simulink model "admire_rtw"  (Simulink 3.00)
settings: Solver=ode3  SolverMode=SingleTasking  StartTime=0.0  StopTime=3000  FixedStep=0.01  RelTol=1e-3  AbsTol=1e-6
values from neighbouring files (symbols this model uses):
  x0 = [ max(eyp,zeros(n,1));max(-eyp,zeros(n,1));zeros(2*m,1)]    [LPwrap.m]
undefined symbols (not defined in the file or in its folder): dalpha_err, dalt_err, dbeta_err, dCl_beta, dCl_dai, dCl_day, dCl_dr, dCl_p, dCl_r, dCm_alpha, dCm_dei, dCm_dey, dCm_dne, dCm_q, dCn_beta, dCn_dna, dCn_dr, dCn_p, dCn_r, dCn_zero, ddc_bw, ddc_rate, ddei_bw, ddei_rate, ddey_bw, ddey_rate, ddle_bw, ddle_rate, ddr_bw, ddr_rate, dIxx, dIxz, dIyy, dIzz, dmass, dVt_err, dxcg, dycg, dzcg, rlimit_c, rlimit_ie, rlimit_le, rlimit_oe, rlimit_r, tasktype, tasktype_pitch, u0corr, u0fcs, u0new, x0diff, y0bare
libraries: simulink_extras x27, simulink3 x22
(part 2 of 2)

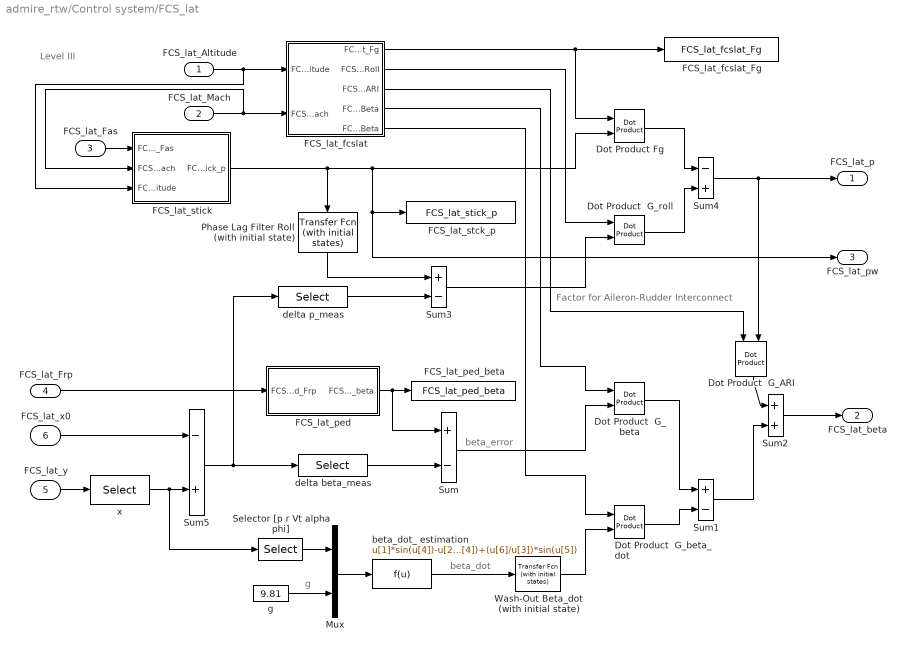
== system admire_rtw/Control system/FCS_lat ==
  note: g
  note: beta_dot
  note: beta_error
  note: Level III
  note: Factor for Aileron-Rudder
      | Interconnect
  "FCS_lat_Altitude " : Inport  Port=1  PortWidth=-1  SampleTime=-1  DataType=auto
      settings: SignalType=auto
  "FCS_lat_Mach " : Inport  Port=2  PortWidth=-1  SampleTime=-1  DataType=auto
      settings: SignalType=auto
  FCS_lat_Fas : Inport  Port=3  PortWidth=-1  SampleTime=-1  DataType=auto
      settings: SignalType=auto
  FCS_lat_Frp : Inport  Port=4  PortWidth=-1  SampleTime=-1  DataType=auto
      settings: SignalType=auto
  "FCS_lat_y " : Inport  Port=5  PortWidth=-1  SampleTime=-1  DataType=auto
      settings: SignalType=auto
  FCS_lat_x0 : Inport  Port=6  PortWidth=-1  SampleTime=-1  DataType=auto
      settings: SignalType=auto
  "  x" : Selector  Elements=[1:12]  InputPortWidth=28
  Dot Product Fg : simulink3/Math/Dot Product
  Dot Product  G_ARI : simulink3/Math/Dot Product  Orientation=down
  Dot Product  G_beta : simulink3/Math/Dot Product
  Dot Product  G_beta_dot : simulink3/Math/Dot Product
  Dot Product  G_roll : simulink3/Math/Dot Product
  FCS_lat_fcslat : Subsystem
      mask Display: disp('Calc of lateral\namplfication\n factors')
  FCS_lat_fcslat_Fg : ToWorkspace  VariableName=FCS_lat_fcslat_Fg  SampleTime=-1  SaveFormat=Matrix
  FCS_lat_ped : Subsystem
      mask Display: disp('FCS lateral pedal\nforce N to beta rad')
  FCS_lat_ped_beta : ToWorkspace  VariableName=FCS_lat_ped_beta  SampleTime=-1  SaveFormat=Matrix
  FCS_lat_stck_p : ToWorkspace  VariableName=FCS_lat_stick_p  SampleTime=-1  SaveFormat=Matrix
  FCS_lat_stick : Subsystem
      mask Display: disp('FCS lateral stick\ngradient\n N to rad/s')
  Mux : Mux  Inputs=2
      settings: DisplayOption=none
  Phase Lag Filter Roll (with initial state) : simulink_extras/Additional Linear/Transfer Fcn (with initial states)  Orientation=down  N=[0 1]  D="[0.25  1]"  X0=x0(39)
  Selector [p r Vt alpha phi] : Selector  Elements=[4 6 1 2 9]  InputPortWidth=12
  Sum : Sum  Inputs=+-  SaturateOnIntegerOverflow=on
  Sum1 : Sum  Inputs=+-  SaturateOnIntegerOverflow=on
  Sum2 : Sum  Inputs=++  SaturateOnIntegerOverflow=on
  Sum3 : Sum  Inputs=+-  SaturateOnIntegerOverflow=on
  Sum4 : Sum  Inputs=-+  SaturateOnIntegerOverflow=on
  Sum5 : Sum  Inputs=-+  SaturateOnIntegerOverflow=on
  Wash-Out Beta_dot (with initial state) : simulink_extras/Additional Linear/Transfer Fcn (with initial states)  N=[5 0]  D="[5  1]"  X0=x0(40)
  beta_dot_ estimation : Fcn  Expr=u[1]*sin(u[4])-u[2]*cos(u[4])+(u[6]/u[3])*sin(u[5])
  delta beta_meas : Selector  Elements=3  InputPortWidth=12
  delta p_meas : Selector  Elements=4  InputPortWidth=12
  g : Constant  Value=9.81
  "FCS_lat_p " : Outport  Port=1  InitialOutput=0
  "FCS_lat_beta " : Outport  Port=2  InitialOutput=0
  FCS_lat_pw : Outport  Port=3  InitialOutput=0
  wires:
  FCS_lat_Fas/1 -> FCS_lat_stick/1("FCS_lat_stick_Fas ")
  Phase Lag Filter Roll (with initial state)/1 -> Sum3/1
  delta p_meas/1 -> Sum3/2
  Mux/1 -> beta_dot_ estimation/1
  Selector [p r Vt alpha phi]/1 -> Mux/1
  g/1 -> Mux/2
  beta_dot_ estimation/1 -> Wash-Out Beta_dot (with initial state)/1
  Sum3/1 -> Dot Product  G_roll/2
  Dot Product  G_roll/1 -> Sum4/2
  Dot Product Fg/1 -> Sum4/1
  Wash-Out Beta_dot (with initial state)/1 -> Dot Product  G_beta_dot/2
  Dot Product  G_beta/1 -> Sum1/1
  Dot Product  G_beta_dot/1 -> Sum1/2
  Sum4/1 -> Dot Product  G_ARI/2, "FCS_lat_p "/1
  Dot Product  G_ARI/1 -> Sum2/1
  Sum2/1 -> "FCS_lat_beta "/1
  Sum1/1 -> Sum2/2
  FCS_lat_stick/1(FCS_lat_stick_p) -> Phase Lag Filter Roll (with initial state)/1, Dot Product Fg/2, FCS_lat_pw/1, FCS_lat_stck_p/1
  FCS_lat_fcslat/2(FCS_lat_fcslat_GRoll) -> Dot Product  G_roll/1
  FCS_lat_fcslat/3(FCS_lat_fcslat_GARI) -> Dot Product  G_ARI/1
  FCS_lat_fcslat/4(FCS_lat_fcslat_GBeta) -> Dot Product  G_beta/1
  FCS_lat_fcslat/5(FCS_lat_fcslat_dGBeta) -> Dot Product  G_beta_dot/1
  delta beta_meas/1 -> Sum/2
  Sum/1 -> Dot Product  G_beta/2
  FCS_lat_Frp/1 -> FCS_lat_ped/1(FCS_lat_ped_Frp)
  "FCS_lat_Altitude "/1 -> FCS_lat_fcslat/1(FCS_lat_fcslat_Altitude), FCS_lat_stick/3("FCS_lat_stick_Altitude ")
  "FCS_lat_Mach "/1 -> FCS_lat_stick/2("FCS_lat_stick_Mach "), FCS_lat_fcslat/2(FCS_lat_fcslat_Mach)
  "FCS_lat_y "/1 -> "  x"/1
  FCS_lat_x0/1 -> Sum5/1
  "  x"/1 -> Sum5/2, Selector [p r Vt alpha phi]/1
  Sum5/1 -> delta beta_meas/1, delta p_meas/1
  FCS_lat_fcslat/1(FCS_lat_fcslat_Fg) -> Dot Product Fg/1, FCS_lat_fcslat_Fg/1
  FCS_lat_ped/1(FCS_lat_ped_beta) -> FCS_lat_ped_beta/1, Sum/1

== system admire_rtw/Control system/FCS_long ==
  note: Level III
  note: q_feedback
      | to integrator
  note: Nz_feedback
      | to integrator
  note: [rad]
  "FCS_long_pw " : Inport  Port=1  PortWidth=-1  SampleTime=-1  DataType=auto
      settings: SignalType=auto
  "FCS_long_Altitude " : Inport  Port=2  PortWidth=-1  SampleTime=-1  DataType=auto
      settings: SignalType=auto
  FCS_long_Mach : Inport  Port=3  PortWidth=-1  SampleTime=-1  DataType=auto
      settings: SignalType=auto
  FCS_long_y : Inport  Port=4  PortWidth=-1  SampleTime=-1  DataType=auto
      settings: SignalType=auto
  FCS_long_Fes : Inport  Port=5  PortWidth=-1  SampleTime=-1  DataType=auto
      settings: SignalType=auto
  "FCS_long_Vt " : Inport  Port=6  PortWidth=-1  SampleTime=-1  DataType=auto
      settings: SignalType=auto
  FCS_long_Nz : Subsystem
      mask Display: disp('FCS_long_Nz')
  FCS_long_qVt : Subsystem
      mask Display: disp('FCS_long_qVt')
  Integrator : Integrator  ExternalReset=none  InitialConditionSource=internal  InitialCondition=x0(38)  LimitOutput=off  UpperSaturationLimit=inf  LowerSaturationLimit=-inf  ShowSaturationPort=off  ShowStatePort=off  AbsoluteTolerance=auto
  Sum : Sum  Inputs=+++  SaturateOnIntegerOverflow=on
  Sum1 : Sum  Inputs=++  SaturateOnIntegerOverflow=on
  FCS_long_x0 : Outport  Port=1  InitialOutput=0
  FCS_long_q : Outport  Port=2  InitialOutput=0
  FCS_long_tss : Outport  Port=3  InitialOutput=0
  wires:
  "FCS_long_Vt "/1 -> FCS_long_qVt/3(FCS_long_qVt_Vt)
  FCS_long_Mach/1 -> FCS_long_qVt/2(FCS_long_qVt_Mach), FCS_long_Nz/2("FCS_long_Nz_Mach ")
  FCS_long_y/1 -> FCS_long_qVt/4(FCS_long_qVt_y), FCS_long_Nz/3(FCS_long_Nz_y)
  FCS_long_qVt/1(FCS_long_qVt_x0) -> FCS_long_x0/1, FCS_long_Nz/5(FCS_long_Nz_x0)
  FCS_long_Fes/1 -> FCS_long_qVt/5(FCS_long_qVt_Fes), FCS_long_Nz/4(FCS_long_Nz_Fes)
  "FCS_long_pw "/1 -> FCS_long_qVt/6("FCS_long_qVt_pw ")
  FCS_long_qVt/2(FCS_long_qVt_tss) -> FCS_long_tss/1
  FCS_long_qVt/3(FCS_long_qVt_q) -> Sum/1
  FCS_long_Nz/1(FCS_long_Nz_control) -> Sum/2
  "FCS_long_Altitude "/1 -> FCS_long_qVt/1(FCS_long_qVt_Altitude), FCS_long_Nz/1("FCS_long_Nz_Altitude ")
  Sum/1 -> FCS_long_q/1
  FCS_long_qVt/4(FCS_long_qVt_fbi) -> Sum1/1
  FCS_long_Nz/2(FCS_long_Nz_fbi) -> Sum1/2
  Integrator/1 -> Sum/3
  Sum1/1 -> Integrator/1

== system admire_rtw/FCS_ae_rl/FCS_ae_rl_lc ==
  note: Level V
  FCS_ae_rl_lc_dlc : Inport  Port=1  PortWidth=-1  SampleTime=-1  DataType=auto
      settings: SignalType=auto
  RL2 : RateLimiter  RisingSlewLimit=rlimit_c+ddc_rate  FallingSlewLimit=-rlimit_c-ddc_rate
  dlc_actuator (with initial state) : simulink_extras/Additional Linear/Transfer Fcn (with initial states)  N=[1]  D="[0.05+ddc_bw  1]"  X0=x0(2)
  dlc_l : ToWorkspace  VariableName=dlc_l  SampleTime=0  SaveFormat=Matrix
  dlc_r : ToWorkspace  VariableName=dlc_r  SampleTime=0  SaveFormat=Matrix
  FCS_ae_rl_lc_dlc_out : Outport  Port=1  InitialOutput=0
  wires:
  FCS_ae_rl_lc_dlc/1 -> dlc_l/1, RL2/1
  dlc_actuator (with initial state)/1 -> FCS_ae_rl_lc_dlc_out/1
  RL2/1 -> dlc_r/1, dlc_actuator (with initial state)/1

== system admire_rtw/FCS_ae_rl/FCS_ae_rl_le ==
  note: Level V
  FCS_ae_rl_le_dle : Inport  Port=1  PortWidth=-1  SampleTime=-1  DataType=auto
      settings: SignalType=auto
  RL2 : RateLimiter  RisingSlewLimit=rlimit_le+ddle_rate  FallingSlewLimit=-rlimit_le-ddle_rate
  dle_actuator (with initial state) : simulink_extras/Additional Linear/Transfer Fcn (with initial states)  N=[1]  D="[0.05+ddle_bw  1]"  X0=x0(8)
  dle_l : ToWorkspace  VariableName=dle_l  SampleTime=0  SaveFormat=Matrix
  dle_r : ToWorkspace  VariableName=dle_r  SampleTime=0  SaveFormat=Matrix
  FCS_ae_rl_le_dle_out : Outport  Port=1  InitialOutput=0
  wires:
  FCS_ae_rl_le_dle/1 -> dle_l/1, RL2/1
  dle_actuator (with initial state)/1 -> FCS_ae_rl_le_dle_out/1
  RL2/1 -> dle_r/1, dle_actuator (with initial state)/1

== system admire_rtw/FCS_ae_rl/FCS_ae_rl_lie ==
  note: Level V
  FCS_ae_rl_lie_dlie : Inport  Port=1  PortWidth=-1  SampleTime=-1  DataType=auto
      settings: SignalType=auto
  RL2 : RateLimiter  RisingSlewLimit=rlimit_ie+ddei_rate  FallingSlewLimit=-rlimit_ie-ddei_rate
  dlie_actuator (with initial state) : simulink_extras/Additional Linear/Transfer Fcn (with initial states)  N=[1]  D="[0.05+ddei_bw  1]"  X0=x0(5)
  dlie_l : ToWorkspace  VariableName=dlie_l  SampleTime=0  SaveFormat=Matrix
  dlie_r : ToWorkspace  VariableName=dlie_r  SampleTime=0  SaveFormat=Matrix
  FCS_ae_rl_lie_dlie_out : Outport  Port=1  InitialOutput=0
  wires:
  dlie_actuator (with initial state)/1 -> FCS_ae_rl_lie_dlie_out/1
  FCS_ae_rl_lie_dlie/1 -> dlie_l/1, RL2/1
  RL2/1 -> dlie_actuator (with initial state)/1, dlie_r/1

== system admire_rtw/FCS_ae_rl/FCS_ae_rl_loe ==
  note: Level V
  FCS_ae_rl_loe_dloe : Inport  Port=1  PortWidth=-1  SampleTime=-1  DataType=auto
      settings: SignalType=auto
  RL2 : RateLimiter  RisingSlewLimit=rlimit_oe+ddey_rate  FallingSlewLimit=-rlimit_oe-ddey_rate
  dloe_actuator (with initial state) : simulink_extras/Additional Linear/Transfer Fcn (with initial states)  N=[1]  D="[0.05+ddey_bw  1]"  X0=x0(6)
  dloe_l : ToWorkspace  VariableName=dloe_l  SampleTime=0  SaveFormat=Matrix
  dloe_r : ToWorkspace  VariableName=dloe_r  SampleTime=0  SaveFormat=Matrix
  FCS_ae_rl_loe_dloe_out : Outport  Port=1  InitialOutput=0
  wires:
  FCS_ae_rl_loe_dloe/1 -> dloe_l/1, RL2/1
  dloe_actuator (with initial state)/1 -> FCS_ae_rl_loe_dloe_out/1
  RL2/1 -> dloe_r/1, dloe_actuator (with initial state)/1

== system admire_rtw/FCS_ae_rl/FCS_ae_rl_r ==
  note: Level V
  FCS_ae_rl_r_dr : Inport  Port=1  PortWidth=-1  SampleTime=-1  DataType=auto
      settings: SignalType=auto
  RL2 : RateLimiter  RisingSlewLimit=rlimit_r+ddr_rate  FallingSlewLimit=-rlimit_r-ddr_rate
  dr_actuator (with initial state) : simulink_extras/Additional Linear/Transfer Fcn (with initial states)  N=[1]  D="[0.05+ddr_bw  1]"  X0=x0(7)
  dr_l : ToWorkspace  VariableName=dr_l  SampleTime=0  SaveFormat=Matrix
  dr_r : ToWorkspace  VariableName=dr_r  SampleTime=0  SaveFormat=Matrix
  FCS_ae_rl_r_dr_out : Outport  Port=1  InitialOutput=0
  wires:
  dr_actuator (with initial state)/1 -> FCS_ae_rl_r_dr_out/1
  FCS_ae_rl_r_dr/1 -> dr_l/1, RL2/1
  RL2/1 -> dr_actuator (with initial state)/1, dr_r/1

== system admire_rtw/FCS_ae_rl/FCS_ae_rl_rc ==
  note: Level V
  FCS_ae_rl_rc_drc : Inport  Port=1  PortWidth=-1  SampleTime=-1  DataType=auto
      settings: SignalType=auto
  RL2 : RateLimiter  RisingSlewLimit=rlimit_c+ddc_rate  FallingSlewLimit=-rlimit_c-ddc_rate
  drc_actuator (with initial state) : simulink_extras/Additional Linear/Transfer Fcn (with initial states)  N=[1]  D="[0.05+ddc_bw  1]"  X0=x0(1)
  drc_l : ToWorkspace  VariableName=drc_l  SampleTime=0  SaveFormat=Matrix
  drc_r : ToWorkspace  VariableName=drc_r  SampleTime=0  SaveFormat=Matrix
  FCS_ae_rl_rc_drc_out : Outport  Port=1  InitialOutput=0
  wires:
  drc_actuator (with initial state)/1 -> FCS_ae_rl_rc_drc_out/1
  FCS_ae_rl_rc_drc/1 -> drc_l/1, RL2/1
  RL2/1 -> drc_actuator (with initial state)/1, drc_r/1

== system admire_rtw/FCS_ae_rl/FCS_ae_rl_rie ==
  note: Level V
  FCS_ae_rl_rie_drie : Inport  Port=1  PortWidth=-1  SampleTime=-1  DataType=auto
      settings: SignalType=auto
  RL2 : RateLimiter  RisingSlewLimit=rlimit_ie+ddei_rate  FallingSlewLimit=-rlimit_ie-ddei_rate
  drie_actuator (with initial state) : simulink_extras/Additional Linear/Transfer Fcn (with initial states)  N=[1]  D="[0.05+ddei_bw  1]"  X0=x0(4)
  drie_l : ToWorkspace  VariableName=drie_l  SampleTime=0  SaveFormat=Matrix
  drie_r : ToWorkspace  VariableName=drie_r  SampleTime=0  SaveFormat=Matrix
  FCS_ae_rl_rie_drie_out : Outport  Port=1  InitialOutput=0
  wires:
  FCS_ae_rl_rie_drie/1 -> drie_l/1, RL2/1
  drie_actuator (with initial state)/1 -> FCS_ae_rl_rie_drie_out/1
  RL2/1 -> drie_r/1, drie_actuator (with initial state)/1

== system admire_rtw/FCS_ae_rl/FCS_ae_rl_roe ==
  note: Level V
  FCS_ae_rl_roe_droe : Inport  Port=1  PortWidth=-1  SampleTime=-1  DataType=auto
      settings: SignalType=auto
  RL2 : RateLimiter  RisingSlewLimit=rlimit_oe+ddey_rate  FallingSlewLimit=-rlimit_oe-ddey_rate
  droe_actuator (with initial state) : simulink_extras/Additional Linear/Transfer Fcn (with initial states)  N=[1]  D="[0.05+ddey_bw  1]"  X0=x0(3)
  droe_l : ToWorkspace  VariableName=droe_l  SampleTime=0  SaveFormat=Matrix
  droe_r : ToWorkspace  VariableName=droe_r  SampleTime=0  SaveFormat=Matrix
  FCS_ae_rl_roe_droe_out : Outport  Port=1  InitialOutput=0
  wires:
  droe_actuator (with initial state)/1 -> FCS_ae_rl_roe_droe_out/1
  FCS_ae_rl_roe_droe/1 -> droe_l/1, RL2/1
  RL2/1 -> droe_actuator (with initial state)/1, droe_r/1

== system admire_rtw/Aircraft response/Sensor models/Subsystem To Gain-Scheduling ==
  note: Level III
  Vt [m/s] : Inport  Port=1  PortWidth=-1  SampleTime=-1  DataType=auto
      settings: SignalType=auto
  alt [m] : Inport  Port=2  PortWidth=-1  SampleTime=-1  DataType=auto
      settings: SignalType=auto
  S-Function : S-Function  FunctionName=machno  PortCounts=[]  SFunctionModules=''
  Mach : Outport  Port=1
  tag scope: Altitude=global, Mach=global
  wires:
  alt [m]/1 -> [Altitude], S-Function/2
  Vt [m/s]/1 -> S-Function/1
  S-Function/1 -> [Mach], Mach/1

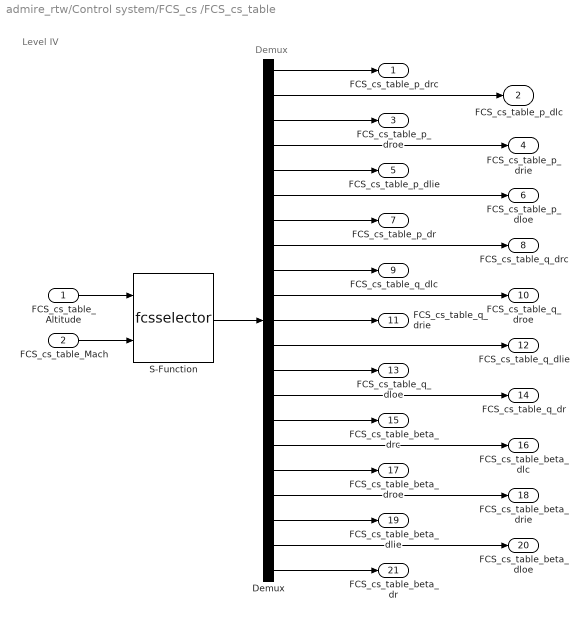
== system admire_rtw/Control system/FCS_cs /FCS_cs_table ==
  note: Level IV
  note: Demux
  FCS_cs_table_Altitude : Inport  Port=1  PortWidth=-1  SampleTime=-1  DataType=auto
      settings: SignalType=auto
  FCS_cs_table_Mach : Inport  Port=2  PortWidth=-1  SampleTime=-1  DataType=auto
      settings: SignalType=auto
  Demux : Demux  Outputs=21
  S-Function : S-Function  FunctionName=fcsselector  PortCounts=[]  SFunctionModules=''
  FCS_cs_table_p_drc : Outport  Port=1
  FCS_cs_table_p_dlc : Outport  Port=2
  FCS_cs_table_p_droe : Outport  Port=3
  FCS_cs_table_p_drie : Outport  Port=4
  FCS_cs_table_p_dlie : Outport  Port=5
  FCS_cs_table_p_dloe : Outport  Port=6
  FCS_cs_table_p_dr : Outport  Port=7
  FCS_cs_table_q_drc : Outport  Port=8
  FCS_cs_table_q_dlc : Outport  Port=9
  FCS_cs_table_q_droe : Outport  Port=10
  FCS_cs_table_q_drie : Outport  Port=11
  FCS_cs_table_q_dlie : Outport  Port=12
  FCS_cs_table_q_dloe : Outport  Port=13
  FCS_cs_table_q_dr : Outport  Port=14
  FCS_cs_table_beta_drc : Outport  Port=15
  FCS_cs_table_beta_dlc : Outport  Port=16
  FCS_cs_table_beta_droe : Outport  Port=17
  FCS_cs_table_beta_drie : Outport  Port=18
  FCS_cs_table_beta_dlie : Outport  Port=19
  FCS_cs_table_beta_dloe : Outport  Port=20
  FCS_cs_table_beta_dr : Outport  Port=21
  wires:
  FCS_cs_table_Altitude/1 -> S-Function/1
  FCS_cs_table_Mach/1 -> S-Function/2
  S-Function/1 -> Demux/1
  Demux/3 -> FCS_cs_table_p_droe/1
  Demux/5 -> FCS_cs_table_p_dlie/1
  Demux/7 -> FCS_cs_table_p_dr/1
  Demux/9 -> FCS_cs_table_q_dlc/1
  Demux/11 -> FCS_cs_table_q_drie/1
  Demux/13 -> FCS_cs_table_q_dloe/1
  Demux/15 -> FCS_cs_table_beta_drc/1
  Demux/17 -> FCS_cs_table_beta_droe/1
  Demux/19 -> FCS_cs_table_beta_dlie/1
  Demux/21 -> FCS_cs_table_beta_dr/1
  Demux/2 -> FCS_cs_table_p_dlc/1
  Demux/4 -> FCS_cs_table_p_drie/1
  Demux/6 -> FCS_cs_table_p_dloe/1
  Demux/8 -> FCS_cs_table_q_drc/1
  Demux/10 -> FCS_cs_table_q_droe/1
  Demux/12 -> FCS_cs_table_q_dlie/1
  Demux/16 -> FCS_cs_table_beta_dlc/1
  Demux/18 -> FCS_cs_table_beta_drie/1
  Demux/20 -> FCS_cs_table_beta_dloe/1
  Demux/14 -> FCS_cs_table_q_dr/1
  Demux/1 -> FCS_cs_table_p_drc/1

== system admire_rtw/Control system/FCS_lat/FCS_lat_fcslat ==
  note: Level IV
  note: S-function
  FCS_lat_fcslat_Altitude : Inport  Port=1  PortWidth=-1  SampleTime=-1  DataType=auto
      settings: SignalType=auto
  FCS_lat_fcslat_Mach : Inport  Port=2  PortWidth=-1  SampleTime=-1  DataType=auto
      settings: SignalType=auto
  S-Function : S-Function  FunctionName=fcslateral  PortCounts=[]  SFunctionModules=''
  FCS_lat_fcslat_Fg : Outport  Port=1
  FCS_lat_fcslat_GRoll : Outport  Port=2
  FCS_lat_fcslat_GARI : Outport  Port=3
  FCS_lat_fcslat_GBeta : Outport  Port=4
  FCS_lat_fcslat_dGBeta : Outport  Port=5
  wires:
  FCS_lat_fcslat_Altitude/1 -> S-Function/1
  FCS_lat_fcslat_Mach/1 -> S-Function/2
  S-Function/1 -> FCS_lat_fcslat_Fg/1
  S-Function/2 -> FCS_lat_fcslat_GBeta/1
  S-Function/3 -> FCS_lat_fcslat_dGBeta/1
  S-Function/4 -> FCS_lat_fcslat_GARI/1
  S-Function/5 -> FCS_lat_fcslat_GRoll/1

== system admire_rtw/Control system/FCS_lat/FCS_lat_ped ==
  note: Level IV
  FCS_lat_ped_Frp : Inport  Port=1  PortWidth=-1  SampleTime=-1  DataType=auto
      settings: SignalType=auto
  Degrees to Radians : simulink_extras/Transformations/Degrees to Radians
  Look-Up Table Frp gradient : Lookup  InputValues=[-200 0 200]  OutputValues=[5 0 -5]
  Saturation : Saturate  UpperLimit=200  LowerLimit=-200
  FCS_lat_ped_beta : Outport  Port=1
  wires:
  Saturation/1 -> Look-Up Table Frp gradient/1
  FCS_lat_ped_Frp/1 -> Saturation/1
  Degrees to Radians/1 -> FCS_lat_ped_beta/1
  Look-Up Table Frp gradient/1 -> Degrees to Radians/1

== system admire_rtw/Control system/FCS_lat/FCS_lat_stick ==
  note: Level IV
  "FCS_lat_stick_Fas " : Inport  Port=1  PortWidth=-1  SampleTime=-1  DataType=auto
      settings: SignalType=auto
  "FCS_lat_stick_Mach " : Inport  Port=2  PortWidth=-1  SampleTime=-1  DataType=auto
      settings: SignalType=auto
  "FCS_lat_stick_Altitude " : Inport  Port=3  PortWidth=-1  SampleTime=-1  DataType=auto
      settings: SignalType=auto
  Dead Zone  +- 3N : DeadZone  LowerValue=-3  UpperValue=3
  Degrees to Radians : simulink_extras/Transformations/Degrees to Radians
  Gain : Gain  Gain=180/80  SaturateOnIntegerOverflow=on
  Saturation : Saturate  UpperLimit=80  LowerLimit=-80
  Terminator : Terminator
  Terminator 2 : Terminator
  FCS_lat_stick_p : Outport  Port=1
  wires:
  Degrees to Radians/1 -> FCS_lat_stick_p/1
  Saturation/1 -> Gain/1
  Gain/1 -> Degrees to Radians/1
  "FCS_lat_stick_Mach "/1 -> Terminator/1
  "FCS_lat_stick_Altitude "/1 -> Terminator 2/1
  Dead Zone  +- 3N/1 -> Saturation/1
  "FCS_lat_stick_Fas "/1 -> Dead Zone  +- 3N/1

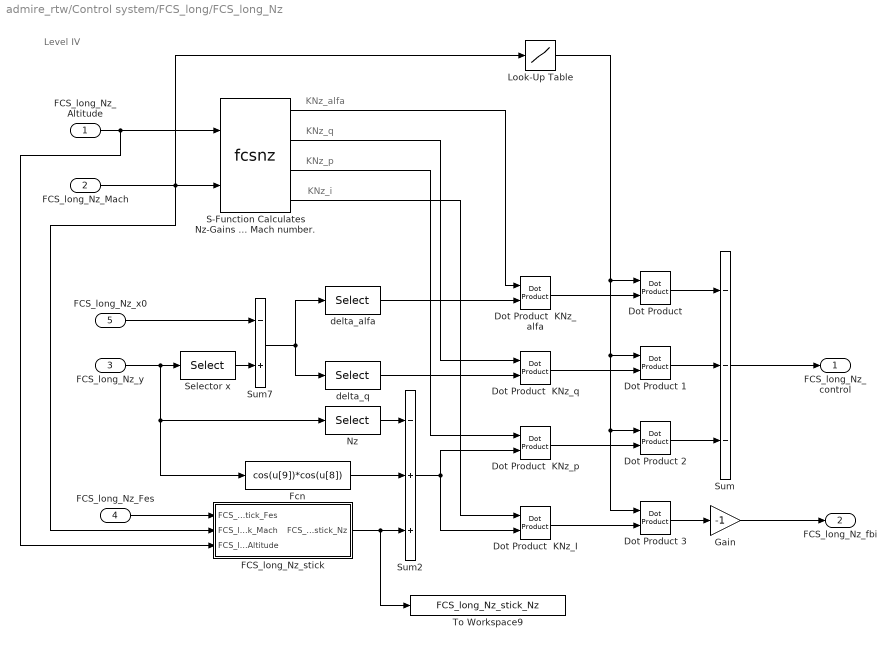
== system admire_rtw/Control system/FCS_long/FCS_long_Nz ==
  note: KNz_alfa
  note: KNz_q
  note: KNz_p
  note: KNz_i
  note: Level IV
  "FCS_long_Nz_Altitude " : Inport  Port=1  PortWidth=-1  SampleTime=-1  DataType=auto
      settings: SignalType=auto
  "FCS_long_Nz_Mach " : Inport  Port=2  PortWidth=-1  SampleTime=-1  DataType=auto
      settings: SignalType=auto
  FCS_long_Nz_y : Inport  Port=3  PortWidth=-1  SampleTime=-1  DataType=auto
      settings: SignalType=auto
  FCS_long_Nz_Fes : Inport  Port=4  PortWidth=-1  SampleTime=-1  DataType=auto
      settings: SignalType=auto
  FCS_long_Nz_x0 : Inport  Port=5  PortWidth=-1  SampleTime=-1  DataType=auto
      settings: SignalType=auto
  Dot Product {,1..3} (4 alike) : simulink3/Math/Dot Product
  Dot Product  KNz_I : simulink3/Math/Dot Product
  Dot Product  KNz_alfa : simulink3/Math/Dot Product
  Dot Product  KNz_p : simulink3/Math/Dot Product
  Dot Product  KNz_q : simulink3/Math/Dot Product
  FCS_long_Nz_stick : Subsystem
      mask Display: disp('FCS_long_Nz_stick')
  Fcn : Fcn  Expr=cos(u[9])*cos(u[8])
  Gain : Gain  Gain=-1  SaturateOnIntegerOverflow=on
  Look-Up Table : Lookup  InputValues=[0 0.58 0.62 2.5]  OutputValues=[0 0 1 1]
  Nz : Selector  Elements=19  InputPortWidth=28
  S-Function Calculates Nz-Gains as a function of altitude and Mach number. : S-Function  FunctionName=fcsnz  PortCounts=[]  SFunctionModules=''
  Selector x : Selector  Elements=[1:12]  InputPortWidth=28
  Sum : Sum  Inputs=---  SaturateOnIntegerOverflow=on
  Sum2 : Sum  Inputs=-++  SaturateOnIntegerOverflow=on
  Sum7 : Sum  Inputs=-+  SaturateOnIntegerOverflow=on
  To Workspace9 : ToWorkspace  VariableName=FCS_long_Nz_stick_Nz  SampleTime=-1  SaveFormat=Matrix
  delta_alfa : Selector  Elements=2  InputPortWidth=12
  delta_q : Selector  Elements=5  InputPortWidth=12
  FCS_long_Nz_control : Outport  Port=1
  FCS_long_Nz_fbi : Outport  Port=2
  wires:
  Nz/1 -> Sum2/1
  FCS_long_Nz_Fes/1 -> FCS_long_Nz_stick/1("FCS_long_Nz_stick_Fes ")
  Selector x/1 -> Sum7/2
  FCS_long_Nz_x0/1 -> Sum7/1
  Sum7/1 -> delta_alfa/1, delta_q/1
  FCS_long_Nz_y/1 -> Selector x/1, Nz/1, Fcn/1
  "FCS_long_Nz_Mach "/1 -> S-Function Calculates Nz-Gains as a function of altitude and Mach number./2, Look-Up Table/1, FCS_long_Nz_stick/2(FCS_long_Nz_stick_Mach)
  Sum2/1 -> Dot Product  KNz_p/2, Dot Product  KNz_I/2
  S-Function Calculates Nz-Gains as a function of altitude and Mach number./4 -> Dot Product  KNz_I/1
  delta_alfa/1 -> Dot Product  KNz_alfa/2
  delta_q/1 -> Dot Product  KNz_q/2
  S-Function Calculates Nz-Gains as a function of altitude and Mach number./3 -> Dot Product  KNz_p/1
  S-Function Calculates Nz-Gains as a function of altitude and Mach number./2 -> Dot Product  KNz_q/1
  S-Function Calculates Nz-Gains as a function of altitude and Mach number./1 -> Dot Product  KNz_alfa/1
  "Dot Product "/1 -> Sum/1
  Dot Product  KNz_alfa/1 -> "Dot Product "/2
  Dot Product 1/1 -> Sum/2
  Dot Product  KNz_q/1 -> Dot Product 1/2
  Look-Up Table/1 -> "Dot Product "/1, Dot Product 1/1, Dot Product 2/1, Dot Product 3/1
  Dot Product 2/1 -> Sum/3
  Dot Product  KNz_p/1 -> Dot Product 2/2
  Dot Product  KNz_I/1 -> Dot Product 3/2
  Sum/1 -> FCS_long_Nz_control/1
  Gain/1 -> FCS_long_Nz_fbi/1
  Dot Product 3/1 -> Gain/1
  "FCS_long_Nz_Altitude "/1 -> S-Function Calculates Nz-Gains as a function of altitude and Mach number./1, FCS_long_Nz_stick/3("FCS_long_Nz_stick_Altitude ")
  FCS_long_Nz_stick/1(FCS_long_Nz_stick_Nz) -> To Workspace9/1, Sum2/3
  Fcn/1 -> Sum2/2

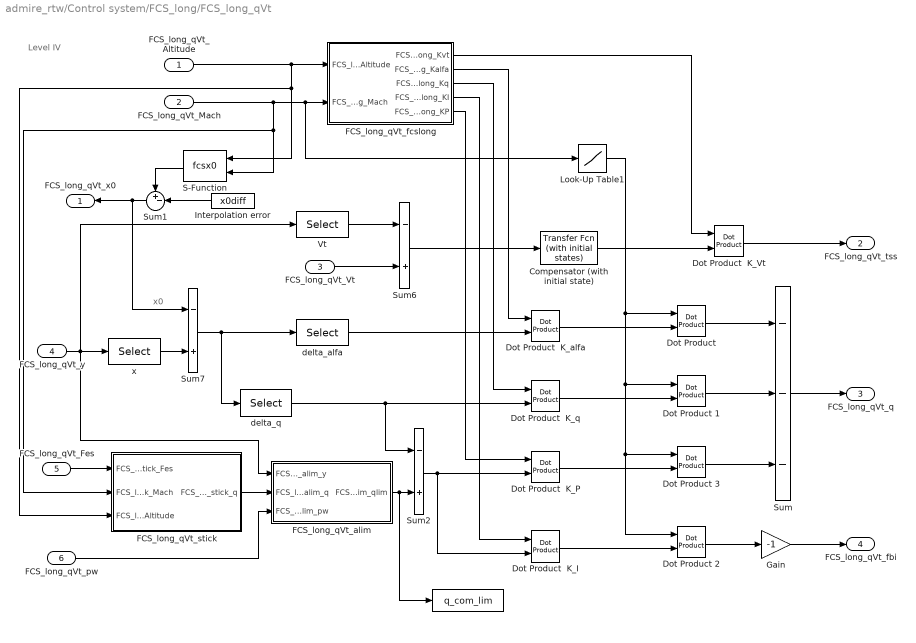
== system admire_rtw/Control system/FCS_long/FCS_long_qVt ==
  note: x0
  note: Level IV
  FCS_long_qVt_Altitude : Inport  Port=1  PortWidth=-1  SampleTime=-1  DataType=auto
      settings: SignalType=auto
  FCS_long_qVt_Mach : Inport  Port=2  PortWidth=-1  SampleTime=-1  DataType=auto
      settings: SignalType=auto
  FCS_long_qVt_Vt : Inport  Port=3  PortWidth=-1  SampleTime=-1  DataType=auto
      settings: SignalType=auto
  FCS_long_qVt_y : Inport  Port=4  PortWidth=-1  SampleTime=-1  DataType=auto
      settings: SignalType=auto
  FCS_long_qVt_Fes : Inport  Port=5  PortWidth=-1  SampleTime=-1  DataType=auto
      settings: SignalType=auto
  "FCS_long_qVt_pw " : Inport  Port=6  PortWidth=-1  SampleTime=-1  DataType=auto
      settings: SignalType=auto
  " " : ToWorkspace  VariableName=q_com_lim  SampleTime=-1  SaveFormat=Matrix
  Compensator (with initial state) : simulink_extras/Additional Linear/Transfer Fcn (with initial states)  N=[15 10]  D="[1  10]"  X0=x0(41)
  Dot Product {,1..3} (4 alike) : simulink3/Math/Dot Product
  Dot Product  K_I : simulink3/Math/Dot Product
  Dot Product  K_P : simulink3/Math/Dot Product
  Dot Product  K_Vt : simulink3/Math/Dot Product
  Dot Product  K_alfa : simulink3/Math/Dot Product
  Dot Product  K_q : simulink3/Math/Dot Product
  FCS_long_qVt_alim : Subsystem
      mask Display: disp('FCS_long_qVt_alim')
  FCS_long_qVt_fcslong : Subsystem
      mask Display: disp('FCS_long_qVt_fcslong')
  FCS_long_qVt_stick : Subsystem
      mask Display: disp('FCS_long_qVt_stick')
  Gain : Gain  Gain=-1  SaturateOnIntegerOverflow=on
  Interpolation error : Constant  Orientation=left  Value=x0diff
  Look-Up Table1 : Lookup  InputValues=[0 0.58 0.62 2.5]  OutputValues=[1 1 0 0]
  S-Function : S-Function  Orientation=left  FunctionName=fcsx0  PortCounts=[]  SFunctionModules=''
  Sum : Sum  Inputs=---  SaturateOnIntegerOverflow=on
  Sum1 : Sum  Orientation=left  Inputs=+-|  SaturateOnIntegerOverflow=on
  Sum2 : Sum  Inputs=-+  SaturateOnIntegerOverflow=on
  Sum6 : Sum  Inputs=-+  SaturateOnIntegerOverflow=on
  Sum7 : Sum  Inputs=-+  SaturateOnIntegerOverflow=on
  Vt : Selector  Elements=1  InputPortWidth=28
  delta_alfa : Selector  Elements=2  InputPortWidth=12
  delta_q : Selector  Elements=5  InputPortWidth=12
  x : Selector  Elements=[1:12]  InputPortWidth=28
  FCS_long_qVt_x0 : Outport  Orientation=left  Port=1
  FCS_long_qVt_tss : Outport  Port=2
  FCS_long_qVt_q : Outport  Port=3
  FCS_long_qVt_fbi : Outport  Port=4
  wires:
  FCS_long_qVt_fcslong/5(FCS_long_qVt_fcslong_KP) -> Dot Product  K_P/1
  FCS_long_qVt_Altitude/1 -> FCS_long_qVt_fcslong/1(FCS_long_qVt_fcslong_Altitude), FCS_long_qVt_stick/3("FCS_long_qVt_stick_Altitude "), S-Function/1
  FCS_long_qVt_Mach/1 -> FCS_long_qVt_stick/2("FCS_long_qVt_stick_Mach "), S-Function/2, FCS_long_qVt_fcslong/2(FCS_long_qVt_fcslong_Mach), Look-Up Table1/1
  delta_alfa/1 -> Dot Product  K_alfa/2
  x/1 -> Sum7/2
  Sum7/1 -> delta_alfa/1, delta_q/1
  delta_q/1 -> Dot Product  K_q/2, Sum2/1
  FCS_long_qVt_y/1 -> x/1, Vt/1, FCS_long_qVt_alim/1(FCS_long_qVt_alim_y)
  FCS_long_qVt_Fes/1 -> FCS_long_qVt_stick/1("FCS_long_qVt_stick_Fes ")
  FCS_long_qVt_alim/1(FCS_long_qVt_alim_qlim) -> Sum2/2, " "/1
  FCS_long_qVt_stick/1("FCS_long_qVt_stick_q ") -> FCS_long_qVt_alim/2("FCS_long_qVt_alim_q ")
  "FCS_long_qVt_pw "/1 -> FCS_long_qVt_alim/3(FCS_long_qVt_alim_pw)
  Compensator (with initial state)/1 -> Dot Product  K_Vt/2
  Dot Product  K_Vt/1 -> FCS_long_qVt_tss/1
  FCS_long_qVt_fcslong/1(FCS_long_qVt_fcslong_Kvt) -> Dot Product  K_Vt/1
  Sum2/1 -> Dot Product  K_P/2, Dot Product  K_I/2
  Dot Product  K_P/1 -> Dot Product 3/2
  Sum/1 -> FCS_long_qVt_q/1
  Dot Product  K_q/1 -> Dot Product 1/2
  Dot Product 1/1 -> Sum/2
  "Dot Product "/1 -> Sum/1
  Dot Product  K_alfa/1 -> "Dot Product "/2
  Look-Up Table1/1 -> "Dot Product "/1, Dot Product 1/1, Dot Product 3/1, Dot Product 2/1
  Sum6/1 -> Compensator (with initial state)/1
  Dot Product 3/1 -> Sum/3
  Gain/1 -> FCS_long_qVt_fbi/1
  Dot Product 2/1 -> Gain/1
  FCS_long_qVt_fcslong/3(FCS_long_qVt_fcslong_Kq) -> Dot Product  K_q/1
  FCS_long_qVt_fcslong/2(FCS_long_qVt_fcslong_Kalfa) -> Dot Product  K_alfa/1
  FCS_long_qVt_Vt/1 -> Sum6/2
  Vt/1 -> Sum6/1
  Dot Product  K_I/1 -> Dot Product 2/2
  FCS_long_qVt_fcslong/4(FCS_long_qVt_fcslong_KI) -> Dot Product  K_I/1
  Interpolation error/1 -> Sum1/2
  S-Function/1 -> Sum1/1
  Sum1/1 -> Sum7/1, FCS_long_qVt_x0/1

== system admire_rtw/Control system/FCS_long/FCS_long_Nz/FCS_long_Nz_stick ==
  note: Level V
  "FCS_long_Nz_stick_Fes " : Inport  Port=1  PortWidth=-1  SampleTime=-1  DataType=auto
      settings: SignalType=auto
  FCS_long_Nz_stick_Mach : Inport  Port=2  PortWidth=-1  SampleTime=-1  DataType=auto
      settings: SignalType=auto
  "FCS_long_Nz_stick_Altitude " : Inport  Port=3  PortWidth=-1  SampleTime=-1  DataType=auto
      settings: SignalType=auto
  Dead Zone  +- 1N : DeadZone  LowerValue=-1  UpperValue=1
  Gain : Gain  Gain=8/80  SaturateOnIntegerOverflow=on
  Saturation [-40,+80]   [Newton] : Saturate  UpperLimit=80  LowerLimit=-40
  Terminator : Terminator
  Terminator 2 : Terminator
  FCS_long_Nz_stick_Nz : Outport  Port=1
  wires:
  Saturation [-40,+80]   [Newton]/1 -> Gain/1
  Gain/1 -> FCS_long_Nz_stick_Nz/1
  "FCS_long_Nz_stick_Altitude "/1 -> Terminator 2/1
  FCS_long_Nz_stick_Mach/1 -> Terminator/1
  Dead Zone  +- 1N/1 -> Saturation [-40,+80]   [Newton]/1
  "FCS_long_Nz_stick_Fes "/1 -> Dead Zone  +- 1N/1

== system admire_rtw/Control system/FCS_long/FCS_long_qVt/FCS_long_qVt_alim ==
  note: Level V
  FCS_long_qVt_alim_y : Inport  Port=1  PortWidth=-1  SampleTime=-1  DataType=auto
      settings: SignalType=auto
  "FCS_long_qVt_alim_q " : Inport  Port=2  PortWidth=-1  SampleTime=-1  DataType=auto
      settings: SignalType=auto
  FCS_long_qVt_alim_pw : Inport  Port=3  PortWidth=-1  SampleTime=-1  DataType=auto
      settings: SignalType=auto
  FCS_long_qVt_alim_nega : Subsystem
      mask Display: disp('FCS_long_qVt_alim\nnegative alpha')
  FCS_long_qVt_alim_posa : Subsystem
      mask Display: disp('FCS_long_qVt_alim\npositive alpha')
  Logical Operator3 : Logic  Operator=OR  Inputs=3
  Logical Operator4 : Logic  Operator=NOT  Inputs=1
  Logical Operator5 : Logic  Orientation=up  Operator=NOT  Inputs=1
  Mach : Fcn  Expr=u[21]
  Product : Product  Inputs=2  SaturateOnIntegerOverflow=on
  Radians to Degrees11 : simulink_extras/Transformations/Radians to Degrees
  Radians to Degrees12 : simulink_extras/Transformations/Radians to Degrees
  Saturation : Saturate  UpperLimit=2.5  LowerLimit=0
  Switch : Switch  Threshold=0.5
  Switch1 : Switch  Threshold=0.5
  alfa : Fcn  Expr=u[2]
  pw demand dead zone : Lookup  InputValues=[-180 -10 -8 8 10 180]  OutputValues=[0 0 0 0 0 0]
  "q dem for zero alpha dot " : Fcn  Expr=(u[4]*cos(u[2])+u[6]*sin(u[2]))*tan(u[3])+(u[19]-cos(u[8])*cos(u[9]))*9.80665*cos(u[2])/(u[1]*cos(u[3]))
  FCS_long_qVt_alim_qlim : Outport  Port=1
  wires:
  Logical Operator3/1 -> Switch/2
  Switch1/1 -> Switch/1
  alfa/1 -> Radians to Degrees11/1
  Mach/1 -> Saturation/1
  Radians to Degrees11/1 -> FCS_long_qVt_alim_posa/2("FCS_long_qVt_alim_posa_alpha "), FCS_long_qVt_alim_nega/2("FCS_long_qVt_alim_nega_alpha ")
  Saturation/1 -> FCS_long_qVt_alim_posa/3("FCS_long_qVt_alim_posa_Mach "), FCS_long_qVt_alim_nega/3("FCS_long_qVt_alim_nega_Mach ")
  FCS_long_qVt_alim_y/1 -> "q dem for zero alpha dot "/1, Mach/1, alfa/1
  "q dem for zero alpha dot "/1 -> FCS_long_qVt_alim_nega/4("FCS_long_qVt_alim_nega_qdem "), FCS_long_qVt_alim_posa/4("FCS_long_qVt_alim_posa_qdem "), Product/1
  "FCS_long_qVt_alim_q "/1 -> FCS_long_qVt_alim_posa/1("FCS_long_qVt_alim_posa_qcom "), FCS_long_qVt_alim_nega/1("FCS_long_qVt_alim_nega_qcom ")
  FCS_long_qVt_alim_nega/2("FCS_long_qVt_alim_nega_q ") -> Switch1/3
  FCS_long_qVt_alim_posa/1(FCS_long_qVt_alim_posa_q) -> Switch1/1
  Logical Operator4/1 -> Switch1/2
  FCS_long_qVt_alim_nega/1(FCS_long_qVt_alim_nega_lim) -> Logical Operator4/1, Logical Operator3/2
  FCS_long_qVt_alim_posa/2(FCS_long_qVt_alim_posa_lim) -> Logical Operator3/1
  Switch/1 -> FCS_long_qVt_alim_qlim/1
  Radians to Degrees12/1 -> pw demand dead zone/1
  Product/1 -> Switch/3
  FCS_long_qVt_alim_pw/1 -> Radians to Degrees12/1
  pw demand dead zone/1 -> Product/2, Logical Operator5/1
  Logical Operator5/1 -> Logical Operator3/3

== system admire_rtw/Control system/FCS_long/FCS_long_qVt/FCS_long_qVt_fcslong ==
  note: Level V
  note: S-function
  FCS_long_qVt_fcslong_Altitude : Inport  Port=1  PortWidth=-1  SampleTime=-1  DataType=auto
      settings: SignalType=auto
  FCS_long_qVt_fcslong_Mach : Inport  Port=2  PortWidth=-1  SampleTime=-1  DataType=auto
      settings: SignalType=auto
  S-Function1 : S-Function  FunctionName=fcslongitudinal  PortCounts=[]  SFunctionModules=''
  FCS_long_qVt_fcslong_Kvt : Outport  Port=1
  FCS_long_qVt_fcslong_Kalfa : Outport  Port=2
  FCS_long_qVt_fcslong_Kq : Outport  Port=3
  FCS_long_qVt_fcslong_KI : Outport  Port=4
  FCS_long_qVt_fcslong_KP : Outport  Port=5
  wires:
  FCS_long_qVt_fcslong_Mach/1 -> S-Function1/2
  FCS_long_qVt_fcslong_Altitude/1 -> S-Function1/1
  S-Function1/1 -> FCS_long_qVt_fcslong_Kalfa/1
  S-Function1/2 -> FCS_long_qVt_fcslong_KI/1
  S-Function1/3 -> FCS_long_qVt_fcslong_KP/1
  S-Function1/4 -> FCS_long_qVt_fcslong_Kq/1
  S-Function1/5 -> FCS_long_qVt_fcslong_Kvt/1

== system admire_rtw/Control system/FCS_long/FCS_long_qVt/FCS_long_qVt_stick ==
  note: Level V
  "FCS_long_qVt_stick_Fes " : Inport  Port=1  PortWidth=-1  SampleTime=-1  DataType=auto
      settings: SignalType=auto
  "FCS_long_qVt_stick_Mach " : Inport  Port=2  PortWidth=-1  SampleTime=-1  DataType=auto
      settings: SignalType=auto
  "FCS_long_qVt_stick_Altitude " : Inport  Port=3  PortWidth=-1  SampleTime=-1  DataType=auto
      settings: SignalType=auto
  " " : ToWorkspace  VariableName=qVt_stick_q_com  SampleTime=-1  SaveFormat=Matrix
  Dead Zone  +- 1N : DeadZone  LowerValue=-1  UpperValue=1
  Degrees to Radians : simulink_extras/Transformations/Degrees to Radians
  Gain : Gain  Gain=22.8083/80  SaturateOnIntegerOverflow=on
  Saturation [-40,+80]   [Newton] : Saturate  UpperLimit=80  LowerLimit=-40
  Terminator : Terminator
  Terminator 2 : Terminator
  "FCS_long_qVt_stick_q " : Outport  Port=1
  wires:
  Gain/1 -> Degrees to Radians/1
  "FCS_long_qVt_stick_Altitude "/1 -> Terminator/1
  "FCS_long_qVt_stick_Mach "/1 -> Terminator 2/1
  Degrees to Radians/1 -> "FCS_long_qVt_stick_q "/1, " "/1
  Saturation [-40,+80]   [Newton]/1 -> Gain/1
  Dead Zone  +- 1N/1 -> Saturation [-40,+80]   [Newton]/1
  "FCS_long_qVt_stick_Fes "/1 -> Dead Zone  +- 1N/1

== system admire_rtw/Control system/FCS_long/FCS_long_qVt/FCS_long_qVt_alim/FCS_long_qVt_alim_nega ==
  note: Level VI
  "FCS_long_qVt_alim_nega_qcom " : Inport  Port=1  PortWidth=-1  SampleTime=-1  DataType=auto
      settings: SignalType=auto
  "FCS_long_qVt_alim_nega_alpha " : Inport  Port=2  PortWidth=-1  SampleTime=-1  DataType=auto
      settings: SignalType=auto
  "FCS_long_qVt_alim_nega_Mach " : Inport  Port=3  PortWidth=-1  SampleTime=-1  DataType=auto
      settings: SignalType=auto
  "FCS_long_qVt_alim_nega_qdem " : Inport  Port=4  PortWidth=-1  SampleTime=-1  DataType=auto
      settings: SignalType=auto
  Look-Up Table1 : Lookup  InputValues=[0 1 1 2.5]  OutputValues=[-8 -8 -3 -3]
  Max : MinMax  Function=max  Inputs=2
  Relational Operator Neg. alpha : RelationalOperator  Operator=<=
  Switch3 : Switch  Threshold=0.5
  FCS_long_qVt_alim_nega_lim : Outport  Port=1
  "FCS_long_qVt_alim_nega_q " : Outport  Port=2
  wires:
  "FCS_long_qVt_alim_nega_Mach "/1 -> Look-Up Table1/1
  Look-Up Table1/1 -> Relational Operator Neg. alpha/2
  "FCS_long_qVt_alim_nega_alpha "/1 -> Relational Operator Neg. alpha/1
  Max/1 -> "FCS_long_qVt_alim_nega_q "/1
  "FCS_long_qVt_alim_nega_qdem "/1 -> Switch3/1
  Relational Operator Neg. alpha/1 -> Switch3/2, FCS_long_qVt_alim_nega_lim/1
  Switch3/1 -> Max/1
  "FCS_long_qVt_alim_nega_qcom "/1 -> Switch3/3, Max/2

== system admire_rtw/Control system/FCS_long/FCS_long_qVt/FCS_long_qVt_alim/FCS_long_qVt_alim_posa ==
  note: Level VI
  "FCS_long_qVt_alim_posa_qcom " : Inport  Port=1  PortWidth=-1  SampleTime=-1  DataType=auto
      settings: SignalType=auto
  "FCS_long_qVt_alim_posa_alpha " : Inport  Port=2  PortWidth=-1  SampleTime=-1  DataType=auto
      settings: SignalType=auto
  "FCS_long_qVt_alim_posa_Mach " : Inport  Port=3  PortWidth=-1  SampleTime=-1  DataType=auto
      settings: SignalType=auto
  "FCS_long_qVt_alim_posa_qdem " : Inport  Port=4  PortWidth=-1  SampleTime=-1  DataType=auto
      settings: SignalType=auto
  Look-Up Table : Lookup  InputValues=[0 0.8 0.8 1 1 1.3 1.3 2.5 ]  OutputValues=[28 28 23 23 18 18 13 13 ]
  Min : MinMax  Function=min  Inputs=2
  Relational Operator Pos. alpha : RelationalOperator  Operator=>=
  Switch2 : Switch  Threshold=0.5
  FCS_long_qVt_alim_posa_q : Outport  Port=1
  FCS_long_qVt_alim_posa_lim : Outport  Port=2
  wires:
  "FCS_long_qVt_alim_posa_alpha "/1 -> Relational Operator Pos. alpha/1
  "FCS_long_qVt_alim_posa_Mach "/1 -> Look-Up Table/1
  Look-Up Table/1 -> Relational Operator Pos. alpha/2
  Relational Operator Pos. alpha/1 -> Switch2/2, FCS_long_qVt_alim_posa_lim/1
  "FCS_long_qVt_alim_posa_qdem "/1 -> Switch2/1
  Min/1 -> FCS_long_qVt_alim_posa_q/1
  Switch2/1 -> Min/1
  "FCS_long_qVt_alim_posa_qcom "/1 -> Switch2/3, Min/2
